simulink model "newtest"  (Simulink 7.9)
settings: Solver=ode45  StartTime=0.0  StopTime=inf  RelTol=1e-3
libraries: utility x1
settings Model: Creator=jorhabib  LastModifiedBy=jorhabib

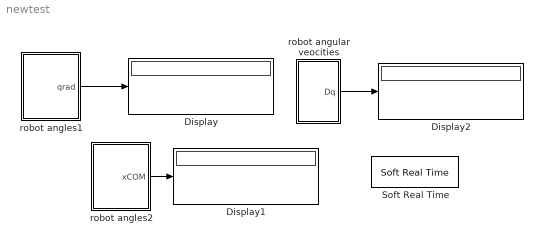
== system newtest ==
  Display : Display
  Display1 : Display
  Display2 : Display
  Soft Real Time : utility/Soft Real Time  x=1
  robot angles1 : Subsystem
  robot angles2 : Subsystem
  robot angular veocities : Subsystem
  wires:
  robot angles1/1(qrad) -> Display/1
  robot angles2/1(xCOM) -> Display1/1
  robot angular veocities/1(Dq) -> Display2/1

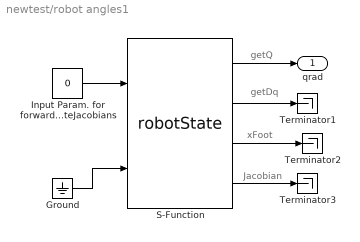
== system newtest/robot angles1 ==
  note: Jacobian
  note: getQ
  note: xFoot
  note: getDq
  Ground : Ground
  "Input Param. for forwardKinematics and  computeJacobians " : Constant  Value=0  OutDataTypeStr=int8
  S-Function : S-Function  FunctionName=robotState  Parameters=val,robotname,localname  EnableBusSupport=off  mask{val=0, robotname='icubSim', localname='robotState'}
      mask prompts: val "Value"; robotname "Robot Name (icub - icubSim)"; localname "Module Name"
  Terminator1 : Terminator
  Terminator2 : Terminator
  Terminator3 : Terminator
  qrad : Outport
  wires:
  S-Function/4 -> Terminator3/1
  "Input Param. for forwardKinematics and  computeJacobians "/1 -> S-Function/1
  S-Function/3 -> Terminator2/1
  S-Function/1 -> qrad/1
  S-Function/2 -> Terminator1/1
  Ground/1 -> S-Function/2

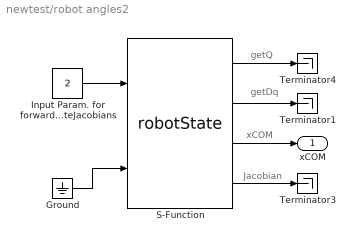
== system newtest/robot angles2 ==
  note: getDq
  note: xCOM
  note: getQ
  note: Jacobian
  Ground : Ground
  "Input Param. for forwardKinematics and  computeJacobians " : Constant  Value=2  OutDataTypeStr=int8
  S-Function : S-Function  FunctionName=robotState  Parameters=val,robotname,localname  EnableBusSupport=off  mask{val=2, robotname='icubSim', localname='robotState'}
      mask prompts: val "Value"; robotname "Robot Name (icub - icubSim)"; localname "Module Name"
  Terminator1 : Terminator
  Terminator3 : Terminator
  Terminator4 : Terminator
  xCOM : Outport
  wires:
  Ground/1 -> S-Function/2
  S-Function/2 -> Terminator1/1
  S-Function/1 -> Terminator4/1
  S-Function/3 -> xCOM/1
  "Input Param. for forwardKinematics and  computeJacobians "/1 -> S-Function/1
  S-Function/4 -> Terminator3/1

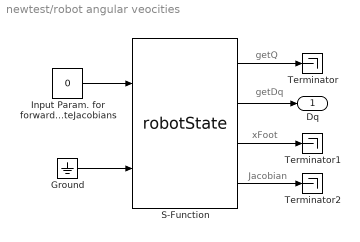
== system newtest/robot angular veocities ==
  note: Jacobian
  note: getQ
  note: xFoot
  note: getDq
  Ground : Ground
  "Input Param. for forwardKinematics and  computeJacobians " : Constant  Value=0  OutDataTypeStr=int8
  S-Function : S-Function  FunctionName=robotState  Parameters=val,robotname,localname  EnableBusSupport=off  mask{val=1, robotname='icubSim', localname='robotState'}
      mask prompts: val "Value"; robotname "Robot Name (icub - icubSim)"; localname "Module Name"
  Terminator : Terminator
  Terminator1 : Terminator
  Terminator2 : Terminator
  Dq : Outport
  wires:
  S-Function/4 -> Terminator2/1
  "Input Param. for forwardKinematics and  computeJacobians "/1 -> S-Function/1
  S-Function/3 -> Terminator1/1
  S-Function/1 -> Terminator/1
  S-Function/2 -> Dq/1
  Ground/1 -> S-Function/2
